simulink model "Energisense"  (R2025a)
settings: Solver=VariableStepAuto  StartTime=0.0  StopTime=100  RelTol=1e-3
settings Model: Creator=Aryan  LastModifiedBy=Aryan

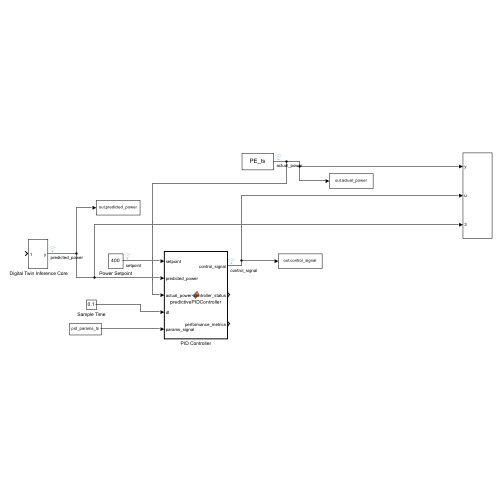
[thumbnail: Simulink's stored preview of the top-level diagram]
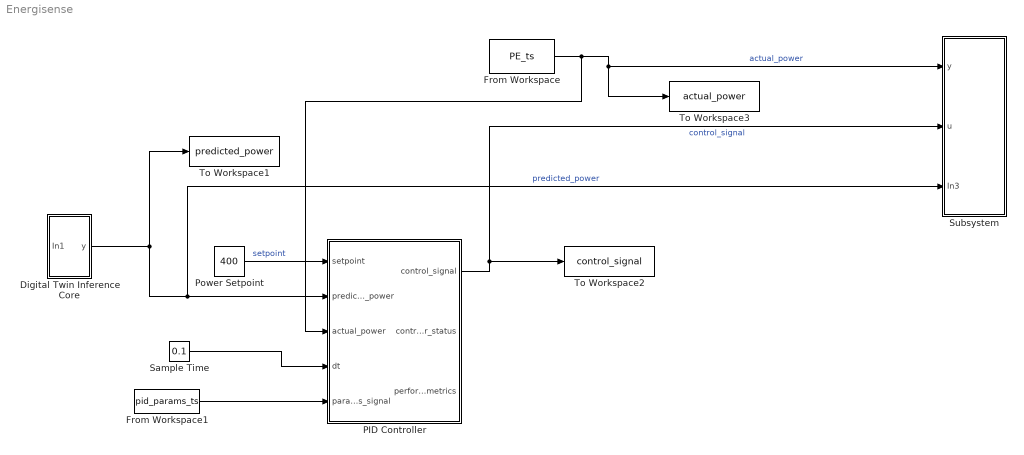
== system Energisense ==
  " Digital Twin Inference Core " : Subsystem
  From Workspace : FromWorkspace  VariableName=PE_ts  OutDataTypeStr=double
  From Workspace1 : FromWorkspace  VariableName=pid_params_ts  OutDataTypeStr=double  SampleTime=0.1
  PID Controller : MATLAB Function  TreatAsAtomicUnit=on
  Power Setpoint : Constant  Value=400
  Sample Time : Constant  Value=0.1
  Subsystem : Subsystem
  To Workspace1 : ToWorkspace  VariableName=predicted_power  SampleTime=-1
  To Workspace2 : ToWorkspace  VariableName=control_signal  SampleTime=-1
  To Workspace3 : ToWorkspace  VariableName=actual_power  SampleTime=-1
  wires:
  Sample Time/1 -> PID Controller/4(dt)
  Power Setpoint/1 -> PID Controller/1(setpoint)  "setpoint"
  " Digital Twin Inference Core "/1(y) -> Subsystem/3(In3), PID Controller/2(predicted_power), To Workspace1/1  "predicted_power"
  PID Controller/1(control_signal) -> Subsystem/2(u), To Workspace2/1  "control_signal"
  From Workspace/1 -> PID Controller/3(actual_power), Subsystem/1(y), To Workspace3/1  "actual_power"
  From Workspace1/1 -> PID Controller/5(params_signal)

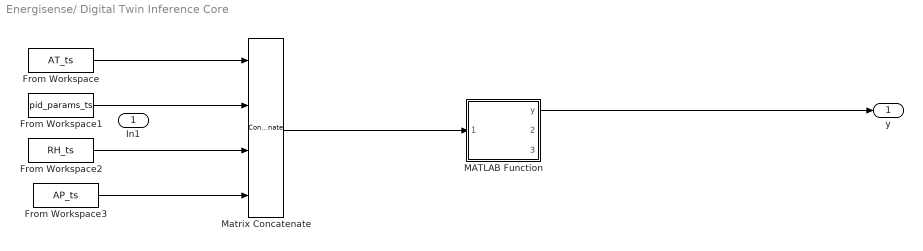
== system Energisense/ Digital Twin Inference Core  ==
  In1 : Inport
  From Workspace : FromWorkspace  VariableName=AT_ts  OutDataTypeStr=double
  From Workspace1 : FromWorkspace  VariableName=pid_params_ts  OutDataTypeStr=double  SampleTime=0.1
  From Workspace2 : FromWorkspace  VariableName=RH_ts  OutDataTypeStr=double
  From Workspace3 : FromWorkspace  VariableName=AP_ts  OutDataTypeStr=double
  MATLAB Function : MATLAB Function  TreatAsAtomicUnit=on
  Matrix Concatenate : Concatenate  NumInputs=4  ConcatenateDimension=2
  y : Outport
  wires:
  Matrix Concatenate/1 -> MATLAB Function/1(input_vector)
  From Workspace2/1 -> Matrix Concatenate/3
  From Workspace1/1 -> Matrix Concatenate/2
  From Workspace/1 -> Matrix Concatenate/1
  MATLAB Function/1(y) -> y/1
  From Workspace3/1 -> Matrix Concatenate/4

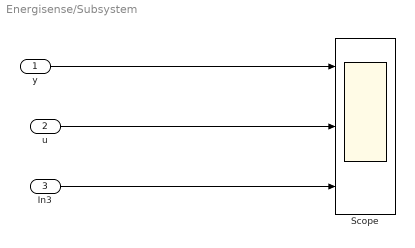
== system Energisense/Subsystem ==
  y : Inport
  u : Inport  Port=2
  In3 : Inport  Port=3
  Scope : Scope  NumInputPorts=3
      settings: Title=Predicted Vs Actual PE  ActiveDisplayYMinimum=-941.66758948423035  ActiveDisplayYMaximum=2122.0302698165196  YLabel=PE  DataLoggingVariableName=Predicted_VS_Actual
  wires:
  y/1 -> Scope/1
  u/1 -> Scope/2
  In3/1 -> Scope/3

== matlab function Energisense/PID Controller ==
  data: setpoint input; predicted_power input; control_signal output; actual_power input; dt input; params_signal input; controller_status output; performance_metrics output
function [control_signal, controller_status, performance_metrics] = predictivePIDController(setpoint, predicted_power, actual_power, dt, params_signal)
%#codegen
% ADVANCED PID CONTROLLER FOR ENERGISENSE - TIME SIGNAL COMPATIBLE
% Updated to work with time signal parameter input for consistency with other inputs
%
% Inputs:
%   setpoint        - Desired power output (MW) [scalar double]
%   predicted_power - Power prediction from Digital Twin (MW) [scalar double]
%   actual_power    - Current actual power (MW) [scalar double] 
%   dt              - Sample time (seconds) [scalar double]
%   params_signal   - Controller parameters time signal [16x1 double vector]
%
% Parameter Signal Order (same as before):
%   1:  Kp                        6:  prediction_weight         11: deadband
%   2:  Ki                        7:  model_quality_threshold   12: adaptive_factor  
%   3:  Kd                        8:  enable_adaptive           13: large_error_threshold
%   4:  u_max                     9:  derivative_filter_alpha   14: small_error_threshold
%   5:  u_min                     10: setpoint_weight           15: feedforward_gain
%                                                               16: disturbance_gain
%
% Outputs:
%   control_signal     - Control signal for power electronics [scalar double]
%   controller_status  - Controller diagnostics [7x1 vector]
%   performance_metrics- Real-time performance metrics [8x1 vector]

%% Input Validation
if nargin < 5
    error('advancedPIDController requires 5 inputs');
end

if ~isscalar(setpoint) || ~isscalar(predicted_power) || ~isscalar(actual_power) || ~isscalar(dt)
    error('All inputs must be scalar values');
end

if dt <= 0
    dt = 0.001;
end

%% Extract Parameters from Time Signal
% params_signal comes as a vector from the From Workspace block
if length(params_signal) >= 16
    % Extract parameters from the current time signal values
    Kp = params_signal(1);
    Ki = params_signal(2);
    Kd = params_signal(3);
    u_max = params_signal(4);
    u_min = params_signal(5);
    prediction_weight = params_signal(6);
    model_quality_threshold = params_signal(7);
    enable_adaptive = logical(params_signal(8) > 0.5);  % Convert to boolean
    derivative_filter_alpha = params_signal(9);
    setpoint_weight = params_signal(10);
    deadband = params_signal(11);
    adaptive_factor = params_signal(12);
    large_error_threshold = params_signal(13);
    small_error_threshold = params_signal(14);
    feedforward_gain = params_signal(15);
    disturbance_gain = params_signal(16);
else
    % Use default parameters if signal is incomplete
    Kp = 1.8; Ki = 0.15; Kd = 0.12;
    u_max = 120.0; u_min = -120.0;
    prediction_weight = 0.6; model_quality_threshold = 0.8;
    enable_adaptive = true; derivative_filter_alpha = 0.2;
    setpoint_weight = 0.9; deadband = 0.5;
    adaptive_factor = 0.02; large_error_threshold = 20.0;
    small_error_threshold = 2.5; feedforward_gain = 0.4;
    disturbance_gain = 0.3;
end

% Additional computed parameters
I_max = u_max * 0.4;  % 40% of max control signal
I_min = u_min * 0.4;  % 40% of min control signal

%% Persistent Variables
persistent integral_error previous_actual_error previous_predicted_error;
persistent previous_setpoint previous_control_signal filtered_derivative;
persistent prediction_error_history adaptive_Kp adaptive_Ki adaptive_Kd initialized;

if isempty(initialized)
    integral_error = 0.0; previous_actual_error = 0.0;
    previous_predicted_error = 0.0; previous_setpoint = 0.0;
    previous_control_signal = 0.0; filtered_derivative = 0.0;
    prediction_error_history = zeros(1, 10);
    adaptive_Kp = Kp; adaptive_Ki = Ki; adaptive_Kd = Kd;
    initialized = true;
end

%% Error Calculations for Predictive Control
% Primary control error: setpoint vs actual power
actual_error = setpoint - actual_power;

% Prediction error: Digital Twin vs actual power
prediction_error = predicted_power - actual_power;

% Predictive error: setpoint vs predicted power
predictive_error = setpoint - predicted_power;

% Apply deadband
if abs(actual_error) < deadband
    actual_error = 0.0;
end

%% Update Prediction Error History
prediction_error_history = [prediction_error_history(2:end), prediction_error];

%% Digital Twin Quality Assessment
prediction_mae = mean(abs(prediction_error_history));
model_quality = exp(-prediction_mae / 5.0);
model_quality = max(0.1, min(1.0, model_quality));

%% Adaptive Gains
current_Kp = adaptive_Kp; current_Ki = adaptive_Ki; current_Kd = adaptive_Kd;

if enable_adaptive
    error_magnitude = abs(actual_error);
    if error_magnitude > large_error_threshold
        current_Kp = min(current_Kp * (1 + adaptive_factor), Kp * 2.0);
        current_Ki = min(current_Ki * (1 + adaptive_factor * 0.5), Ki * 1.5);
    elseif error_magnitude < small_error_threshold
        current_Kp = max(current_Kp * (1 - adaptive_factor * 0.5), Kp * 0.5);
        current_Ki = max(current_Ki * (1 - adaptive_factor * 0.3), Ki * 0.5);
    end
end

% Model quality adaptation
if model_quality > model_quality_threshold
    current_Kp = current_Kp * 0.8;  % More predictive
else
    current_Kp = current_Kp * 1.2;  % More reactive
end

%% PID Terms with Predictive Elements
% Proportional term: weighted combination
P_actual = current_Kp * actual_error;
P_predictive = current_Kp * predictive_error * prediction_weight;
P_term = P_actual * (1.0 - prediction_weight) + P_predictive * prediction_weight;

% Integral term
I_term = current_Ki * integral_error;

% Derivative term with filtering
D_term = 0.0;
if dt > 0
    actual_derivative = (actual_error - previous_actual_error) / dt;
    predictive_derivative = (predictive_error - previous_predicted_error) / dt;
    combined_derivative = actual_derivative * (1.0 - prediction_weight) + predictive_derivative * prediction_weight;
    
    % Apply derivative filtering
    filtered_derivative = derivative_filter_alpha * combined_derivative + (1.0 - derivative_filter_alpha) * filtered_derivative;
    D_term = current_Kd * filtered_derivative;
end

%% Feed-forward Control
feedforward_term = 0.0;
if dt > 0
    prediction_ff = (setpoint - predicted_power) * feedforward_gain * model_quality;
    setpoint_rate = (setpoint - previous_setpoint) / dt;
    rate_ff = setpoint_rate * feedforward_gain * 0.5;
    feedforward_term = prediction_ff + rate_ff;
end

%% Disturbance Compensation
disturbance_compensation = 0.0;
recent_errors = prediction_error_history(end-4:end);
persistent_bias = mean(recent_errors);
if abs(persistent_bias) > 2.0 && std(recent_errors) < abs(persistent_bias) * 0.5
    disturbance_compensation = -persistent_bias * disturbance_gain;
end

%% Total Control Signal
raw_control_signal = P_term + I_term + D_term + feedforward_term + disturbance_compensation;
control_signal = max(u_min, min(raw_control_signal, u_max));

%% Anti-Windup with Prediction Awareness
is_saturated = (control_signal ~= raw_control_signal);
integrate_condition = true;
if is_saturated && sign(actual_error) == sign(integral_error)
    integrate_condition = false;
end
if model_quality > model_quality_threshold && sign(predictive_error) ~= sign(actual_error)
    integrate_condition = true;
end
if integrate_condition
    integral_error = integral_error + actual_error * dt;
end
integral_error = max(I_min, min(integral_error, I_max));

%% Update Persistent Variables
previous_actual_error = actual_error;
previous_predicted_error = predictive_error;
previous_setpoint = setpoint;
previous_control_signal = control_signal;
alpha = 0.001;
adaptive_Kp = current_Kp * alpha + adaptive_Kp * (1.0 - alpha);
adaptive_Ki = current_Ki * alpha + adaptive_Ki * (1.0 - alpha);
adaptive_Kd = current_Kd * alpha + adaptive_Kd * (1.0 - alpha);

%% Generate Outputs
% Controller Status (7x1 vector for Simulink compatibility)
controller_status = [
    current_Kp;           % Current proportional gain
    current_Ki;           % Current integral gain
    current_Kd;           % Current derivative gain
    model_quality;        % Digital Twin quality (0-1)
    prediction_error;     % Current prediction error (MW)
    integral_error;       % Current integral value
    model_quality         % Controller health metric
];

% Performance Metrics (8x1 vector for Simulink compatibility)
control_effort = abs(control_signal);
prediction_accuracy = model_quality * 100;
if abs(setpoint) > 1.0
    tracking_efficiency = (1.0 - abs(actual_error) / abs(setpoint)) * 100;
else
    tracking_efficiency = 100.0;
end
tracking_efficiency = max(0, min(100, tracking_efficiency));

performance_metrics = [
    actual_error;                    % Current tracking error (MW)
    abs(actual_error);              % Absolute tracking error (MW)
    abs(prediction_error);          % Absolute prediction error (MW)
    model_quality;                  % Digital Twin quality (0-1)
    control_effort;                 % Control signal magnitude
    prediction_accuracy;            % Prediction accuracy (%)
    tracking_efficiency;            % Tracking efficiency (%)
    1.0                             % Sample indicator
];

end

== matlab function Energisense/ Digital Twin Inference Core /MATLAB Function ==
  data: input_vector input; y output; confidence output; anomaly_flag output
function [y, confidence, anomaly_flag] = fcn(input_vector)
%#codegen
% Digital Twin - Complete CCPP Model with Bias Correction

    % Extract scalars from input vector
    if numel(input_vector) >= 4
        AT = double(input_vector(1));  % Ambient Temperature
        V = double(input_vector(2));   % Vacuum
        RH = double(input_vector(3));  % Relative Humidity  
        AP = double(input_vector(4));  % Atmospheric Pressure
    else
        % Default values if input is wrong size
        AT = 20.0;
        V = 40.0;
        RH = 70.0;
        AP = 1013.0;
    end
    
    % Input validation
    input_valid = true;
    if isnan(AT) || isnan(V) || isnan(RH) || isnan(AP) || ...
       isinf(AT) || isinf(V) || isinf(RH) || isinf(AP) || ...
       (AT < -50.0) || (AT > 100.0) || (V < 0.0) || (V > 200.0) || ...
       (RH < 0.0) || (RH > 150.0) || (AP < 900.0) || (AP > 1100.0)
        input_valid = false;
    end
    
    if input_valid
        % COMPLETE CCPP PHYSICS MODEL
        base_power = 454.5;
        
        % Primary linear effects (most important)
        temp_effect = -2.2 * AT;       % Temperature impact
        vacuum_effect = -0.39 * V;     % Vacuum impact  
        humidity_effect = -0.078 * RH; % Humidity impact
        pressure_effect = 0.043 * AP;  % Pressure impact
        
        % Interaction effects (ensemble model characteristics)
        AT_V_int = 0.0086 * AT * V;
        AT_RH_int = 0.0021 * AT * RH;
        V_RH_int = 0.0012 * V * RH;
        AT_AP_int = 0.0018 * AT * AP;
        
        % Non-linear effects (polynomial terms)
        AT_sq = -0.0189 * AT * AT;
        V_sq = -0.0067 * V * V;
        RH_sq = -0.0003 * RH * RH;
        
        % Higher-order interactions (ensemble specialty)
        three_way_1 = 0.000043 * AT * V * RH;
        three_way_2 = 0.000028 * AT * V * AP;
        
        % Threshold effects (decision tree characteristics)
        threshold_adj = 0.0;
        if AT > 20.0
            threshold_adj = threshold_adj - 0.5 * (AT - 20.0);
        end
        if V > 50.0
            threshold_adj = threshold_adj - 0.3 * (V - 50.0);
        end
        
        % FIXED BIAS CORRECTION (was 2.0, now 27.0)
        bias_correction = 27.0;  % Corrects the 26.4 MW systematic error
        
        % Calculate total power output
        y = base_power + temp_effect + vacuum_effect + humidity_effect + pressure_effect + ...
            AT_V_int + AT_RH_int + V_RH_int + AT_AP_int + ...
            AT_sq + V_sq + RH_sq + three_way_1 + three_way_2 + ...
            threshold_adj + bias_correction;
        
        % DYNAMIC CONFIDENCE CALCULATION
        % Higher confidence when closer to optimal conditions
        AT_optimal = 15.0;
        V_optimal = 40.0; 
        RH_optimal = 60.0;
        AP_optimal = 1013.0;
        
        % Operating ranges for confidence calculation
        AT_range = 35.3;  % Full operating range
        V_range = 56.2;
        RH_range = 74.6;
        AP_range = 40.41;
        
        % Distance-based confidence (closer to optimal = higher confidence)
        AT_conf = 1.0 - 0.8 * abs(AT - AT_optimal) / AT_range;
        V_conf = 1.0 - 0.6 * abs(V - V_optimal) / V_range;
        RH_conf = 1.0 - 0.3 * abs(RH - RH_optimal) / RH_range;
        AP_conf = 1.0 - 0.2 * abs(AP - AP_optimal) / AP_range;
        
        % Weighted confidence (AT and V most important in CCPP)
        confidence = 0.4 * AT_conf + 0.3 * V_conf + 0.2 * RH_conf + 0.1 * AP_conf;
        
        % ANOMALY DETECTION - check operating envelope
        AT_ok = (AT >= 1.81) && (AT <= 37.11);
        V_ok = (V >= 25.36) && (V <= 81.56);
        RH_ok = (RH >= 25.56) && (RH <= 100.16);
        AP_ok = (AP >= 992.89) && (AP <= 1033.30);
        
        anomaly_flag = ~(AT_ok && V_ok && RH_ok && AP_ok);
        
        % Reduce confidence if anomaly detected
        if anomaly_flag
            confidence = confidence * 0.5;
        end
        
    else
        % Invalid inputs - safe defaults
        y = 450.0;
        confidence = 0.1;
        anomaly_flag = true;
    end
    
    % Final bounds and type conversion
    y = max(400.0, min(500.0, y));
    confidence = max(0.1, min(1.0, confidence));
    
    % Ensure scalar outputs for Simulink
    y = double(y);
    confidence = double(confidence);
    anomaly_flag = logical(anomaly_flag);
end
